simulink model "A"  (R2017b)
settings: Solver=VariableStepAuto  StartTime=0.0  StopTime=10  RelTol=1e-3
libraries: dspsigops x2, simulink_extras x1
settings Model: Creator=Joss  LastModifiedBy=Joss

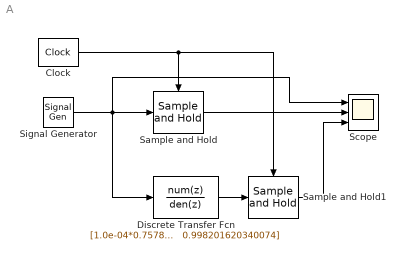
== system A ==
  Clock : simulink_extras/Flip Flops/Clock  period=0.1
  Discrete Transfer Fcn : DiscreteTransferFcn  Numerator="[1.0e-04*0.757817206696876   1.0e-04*0.036966693011120  1.0e-04*-0.720850513687976]"  Denominator="[1.000000000000000  -1.998197623940829   0.998201620340074]"
  Sample and Hold : dspsigops/Sample and Hold  trig=Rising edge  initCond=0  latchinput=off
  Sample and Hold1 : dspsigops/Sample and Hold  trig=Rising edge  initCond=0  latchinput=off
  Scope : Scope  NumInputPorts=3
  Signal Generator : SignalGenerator  VectorParams1D=off
  wires:
  Clock/1 -> Sample and Hold/Trigger, Sample and Hold1/Trigger
  Discrete Transfer Fcn/1 -> Sample and Hold1/1
  Signal Generator/1 -> Scope/1, Discrete Transfer Fcn/1, Sample and Hold/1
  Sample and Hold1/1 -> Scope/3
  Sample and Hold/1 -> Scope/2
